simulink model "E3_1_Desequilibrio"  (R2018a)
settings: Solver=VariableStepAuto  StartTime=0.0  StopTime=0.5  RelTol=1e-3
libraries: powerlib x73, powerlib_meascontrol x36
settings Model: Creator=Rafael Pavan  LastModifiedBy=Rafael Pavan

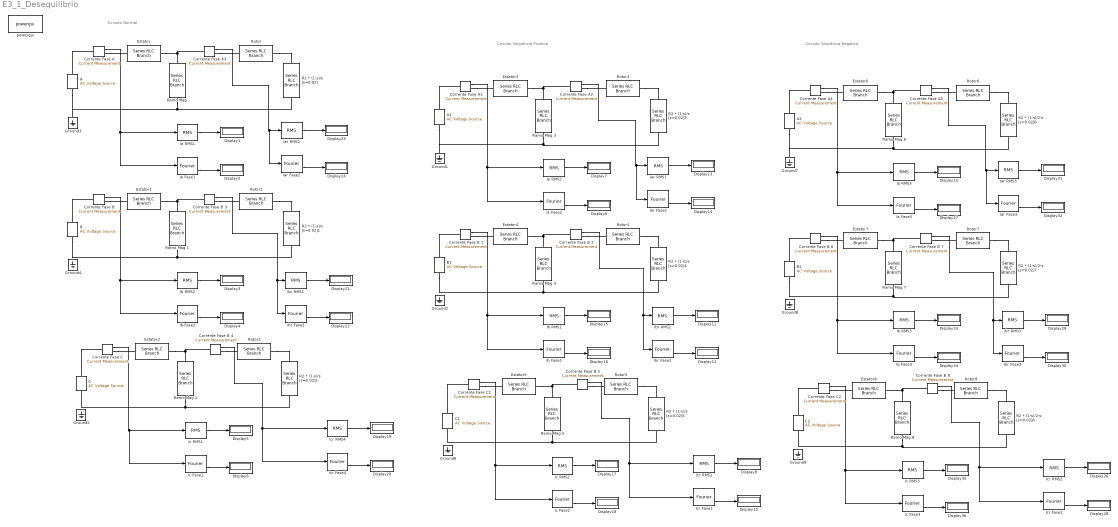
== system E3_1_Desequilibrio ==
  note: Circuito Normal
  note: Circuito Sequência Positiva
  note: Circuito Sequência Negativa
  A : powerlib/Electrical Sources/AC Voltage Source  Amplitude=171.26  Phase=0  Frequency=60  SampleTime=0  Measurements=None  BusType=PV  Pref=100e4  Qref=0  Qmin=-inf  Qmax=+inf
  A1 : powerlib/Electrical Sources/AC Voltage Source  Amplitude=179.5550  Phase=0  Frequency=60  SampleTime=0  Measurements=None  BusType=PV  Pref=100e4  Qref=0  Qmin=-inf  Qmax=+inf
  A2 : powerlib/Electrical Sources/AC Voltage Source  Amplitude=4.7693  Phase=-150.3406  Frequency=60  SampleTime=0  Measurements=None  BusType=PV  Pref=100e4  Qref=0  Qmin=-inf  Qmax=+inf
  B : powerlib/Electrical Sources/AC Voltage Source  Amplitude=179.605  Phase=-120  Frequency=60  SampleTime=0  Measurements=None  BusType=PV  Pref=100e4  Qref=0  Qmin=-inf  Qmax=+inf
  B1 : powerlib/Electrical Sources/AC Voltage Source  Amplitude=179.5550  Phase=-120  Frequency=60  SampleTime=0  Measurements=None  BusType=PV  Pref=100e4  Qref=0  Qmin=-inf  Qmax=+inf
  B2 : powerlib/Electrical Sources/AC Voltage Source  Amplitude=4.7693  Phase=-30.3441  Frequency=60  SampleTime=0  Measurements=None  BusType=PV  Pref=100e4  Qref=0  Qmin=-inf  Qmax=+inf
  C : powerlib/Electrical Sources/AC Voltage Source  Amplitude=187.80  Phase=120  Frequency=60  SampleTime=0  Measurements=None  BusType=PV  Pref=100e4  Qref=0  Qmin=-inf  Qmax=+inf
  C1 : powerlib/Electrical Sources/AC Voltage Source  Amplitude=179.5550  Phase=120  Frequency=60  SampleTime=0  Measurements=None  BusType=PV  Pref=100e4  Qref=0  Qmin=-inf  Qmax=+inf
  C2 : powerlib/Electrical Sources/AC Voltage Source  Amplitude=4.7693  Phase=89.6524  Frequency=60  SampleTime=0  Measurements=None  BusType=PV  Pref=100e4  Qref=0  Qmin=-inf  Qmax=+inf
  Corrente Fase A{,1..5} (6 alike) : powerlib/Measurements/Current Measurement  PhasorSimulation=off  OutputType=Complex  PSBequivalent=0
  Corrente Fase B {,1..8} (9 alike) : powerlib/Measurements/Current Measurement  PhasorSimulation=off  OutputType=Complex  PSBequivalent=0
  Corrente Fase C : powerlib/Measurements/Current Measurement  PhasorSimulation=off  OutputType=Complex  PSBequivalent=0
  Corrente Fase C1 : powerlib/Measurements/Current Measurement  PhasorSimulation=off  OutputType=Complex  PSBequivalent=0
  Corrente Fase C2 : powerlib/Measurements/Current Measurement  PhasorSimulation=off  OutputType=Complex  PSBequivalent=0
  Display{1..36} (36 alike) : Display
  Estator{,1..8} (9 alike) : powerlib/Elements/Series RLC Branch  LConnTagsString=__new0  RConnTagsString=__new0  BranchType=RL  Resistance=0.294  Inductance=1.33428e-3  SetiL0=off  InitialCurrent=0  Capacitance=1e-6  Setx0=off  InitialVoltage=0  Measurements=None
  Ground{1..9} (9 alike) : powerlib/Elements/Ground  LConnTagsString=a
  Ia Fase1 : powerlib_meascontrol/Measurements/Fourier  Freq=60  n=1  InInit=[0, 0]  Ts=0
      settings: SourceProductName=Simscape Power Systems
  Ia Fase2 : powerlib_meascontrol/Measurements/Fourier  Freq=60  n=1  InInit=[0, 0]  Ts=0
      settings: SourceProductName=Simscape Power Systems
  Ia Fase3 : powerlib_meascontrol/Measurements/Fourier  Freq=60  n=1  InInit=[0, 0]  Ts=0
      settings: SourceProductName=Simscape Power Systems
  Ia RMS1 : powerlib_meascontrol/Measurements/RMS  TrueRMS=on  Freq=60  RMSInit=120  Ts=0
  Ia RMS2 : powerlib_meascontrol/Measurements/RMS  TrueRMS=on  Freq=60  RMSInit=120  Ts=0
  Ia RMS3 : powerlib_meascontrol/Measurements/RMS  TrueRMS=on  Freq=60  RMSInit=120  Ts=0
  Iar Fase1 : powerlib_meascontrol/Measurements/Fourier  Freq=60  n=1  InInit=[0, 0]  Ts=0
      settings: SourceProductName=Simscape Power Systems
  Iar Fase2 : powerlib_meascontrol/Measurements/Fourier  Freq=60  n=1  InInit=[0, 0]  Ts=0
      settings: SourceProductName=Simscape Power Systems
  Iar Fase3 : powerlib_meascontrol/Measurements/Fourier  Freq=60  n=1  InInit=[0, 0]  Ts=0
      settings: SourceProductName=Simscape Power Systems
  Iar RMS1 : powerlib_meascontrol/Measurements/RMS  TrueRMS=on  Freq=60  RMSInit=120  Ts=0
  Iar RMS2 : powerlib_meascontrol/Measurements/RMS  TrueRMS=on  Freq=60  RMSInit=120  Ts=0
  Iar RMS3 : powerlib_meascontrol/Measurements/RMS  TrueRMS=on  Freq=60  RMSInit=120  Ts=0
  Ib Fase1 : powerlib_meascontrol/Measurements/Fourier  Freq=60  n=1  InInit=[0, 0]  Ts=0
      settings: SourceProductName=Simscape Power Systems
  Ib Fase2 : powerlib_meascontrol/Measurements/Fourier  Freq=60  n=1  InInit=[0, 0]  Ts=0
      settings: SourceProductName=Simscape Power Systems
  Ib Fase3 : powerlib_meascontrol/Measurements/Fourier  Freq=60  n=1  InInit=[0, 0]  Ts=0
      settings: SourceProductName=Simscape Power Systems
  Ib RMS1 : powerlib_meascontrol/Measurements/RMS  TrueRMS=on  Freq=60  RMSInit=120  Ts=0
  Ib RMS2 : powerlib_meascontrol/Measurements/RMS  TrueRMS=on  Freq=60  RMSInit=120  Ts=0
  Ib RMS3 : powerlib_meascontrol/Measurements/RMS  TrueRMS=on  Freq=60  RMSInit=120  Ts=0
  Ibr Fase1 : powerlib_meascontrol/Measurements/Fourier  Freq=60  n=1  InInit=[0, 0]  Ts=0
      settings: SourceProductName=Simscape Power Systems
  Ibr Fase2 : powerlib_meascontrol/Measurements/Fourier  Freq=60  n=1  InInit=[0, 0]  Ts=0
      settings: SourceProductName=Simscape Power Systems
  Ibr Fase3 : powerlib_meascontrol/Measurements/Fourier  Freq=60  n=1  InInit=[0, 0]  Ts=0
      settings: SourceProductName=Simscape Power Systems
  Ibr RMS1 : powerlib_meascontrol/Measurements/RMS  TrueRMS=on  Freq=60  RMSInit=120  Ts=0
  Ibr RMS2 : powerlib_meascontrol/Measurements/RMS  TrueRMS=on  Freq=60  RMSInit=120  Ts=0
  Ibr RMS3 : powerlib_meascontrol/Measurements/RMS  TrueRMS=on  Freq=60  RMSInit=120  Ts=0
  Ic Fase1 : powerlib_meascontrol/Measurements/Fourier  Freq=60  n=1  InInit=[0, 0]  Ts=0
      settings: SourceProductName=Simscape Power Systems
  Ic Fase2 : powerlib_meascontrol/Measurements/Fourier  Freq=60  n=1  InInit=[0, 0]  Ts=0
      settings: SourceProductName=Simscape Power Systems
  Ic Fase3 : powerlib_meascontrol/Measurements/Fourier  Freq=60  n=1  InInit=[0, 0]  Ts=0
      settings: SourceProductName=Simscape Power Systems
  Ic RMS1 : powerlib_meascontrol/Measurements/RMS  TrueRMS=on  Freq=60  RMSInit=120  Ts=0
  Ic RMS2 : powerlib_meascontrol/Measurements/RMS  TrueRMS=on  Freq=60  RMSInit=120  Ts=0
  Ic RMS3 : powerlib_meascontrol/Measurements/RMS  TrueRMS=on  Freq=60  RMSInit=120  Ts=0
  Icr Fase1 : powerlib_meascontrol/Measurements/Fourier  Freq=60  n=1  InInit=[0, 0]  Ts=0
      settings: SourceProductName=Simscape Power Systems
  Icr Fase2 : powerlib_meascontrol/Measurements/Fourier  Freq=60  n=1  InInit=[0, 0]  Ts=0
      settings: SourceProductName=Simscape Power Systems
  Icr Fase4 : powerlib_meascontrol/Measurements/Fourier  Freq=60  n=1  InInit=[0, 0]  Ts=0
      settings: SourceProductName=Simscape Power Systems
  Icr RMS1 : powerlib_meascontrol/Measurements/RMS  TrueRMS=on  Freq=60  RMSInit=120  Ts=0
  Icr RMS2 : powerlib_meascontrol/Measurements/RMS  TrueRMS=on  Freq=60  RMSInit=120  Ts=0
  Icr RMS4 : powerlib_meascontrol/Measurements/RMS  TrueRMS=on  Freq=60  RMSInit=120  Ts=0
  R2 * (1-s)/2-s [s=0.02]6 : powerlib/Elements/Series RLC Branch  LConnTagsString=__new0  RConnTagsString=__new0  BranchType=R  Resistance=0.2489  Inductance=1e-3  SetiL0=off  InitialCurrent=0  Capacitance=1e-6  Setx0=off  InitialVoltage=0  Measurements=None
  R2 * (1-s)/2-s [s=0.02]7 : powerlib/Elements/Series RLC Branch  LConnTagsString=__new0  RConnTagsString=__new0  BranchType=R  Resistance=0.2489  Inductance=1e-3  SetiL0=off  InitialCurrent=0  Capacitance=1e-6  Setx0=off  InitialVoltage=0  Measurements=None
  R2 * (1-s)/2-s [s=0.02]8 : powerlib/Elements/Series RLC Branch  LConnTagsString=__new0  RConnTagsString=__new0  BranchType=R  Resistance=0.2489  Inductance=1e-3  SetiL0=off  InitialCurrent=0  Capacitance=1e-6  Setx0=off  InitialVoltage=0  Measurements=None
  R2 * (1-s)/s [s=0.02]{,1..5} (6 alike) : powerlib/Elements/Series RLC Branch  LConnTagsString=__new0  RConnTagsString=__new0  BranchType=R  Resistance=24.647  Inductance=1e-3  SetiL0=off  InitialCurrent=0  Capacitance=1e-6  Setx0=off  InitialVoltage=0  Measurements=None
  Ramo Mag.{,1..8} (9 alike) : powerlib/Elements/Series RLC Branch  LConnTagsString=__new0  RConnTagsString=__new0  BranchType=L  Resistance=1  Inductance=0.0351477  SetiL0=off  InitialCurrent=0  Capacitance=1e-6  Setx0=off  InitialVoltage=0  Measurements=None
  Rotor{,1..8} (9 alike) : powerlib/Elements/Series RLC Branch  LConnTagsString=__new0  RConnTagsString=__new0  BranchType=RL  Resistance=0.503  Inductance=0.554406e-3  SetiL0=off  InitialCurrent=0  Capacitance=1e-6  Setx0=off  InitialVoltage=0  Measurements=None
  powergui : powerlib/powergui  Priority=1  SimulationMode=Continuous  SampleTime=50e-6  frequency=60  Iterations=50  frequencyindice=60  Pbase=100e6  ErrMax=1e-4  UnitsV=kV  UnitsW=MW  buscounter=0  FunctionMessages=on  echomessages=off  EnableUseOfTLC=off  CurrentSourceSwitches=off  DisableSnubberDevices=off  DisableRonSwitches=off  DisableVfSwitches=off  DisplayEquations=off  SolverType=Tustin/Backward Euler (TBE)  Interpol=off  ExternalGateDelay=off  methode=off  Ts=100  x0status=blocks  SPID=on  SwTol=0  HookPort=off  RestoreLinks=warning  ResistiveCurrentMeasurement=off  Frange=[0:2:500]  Ylog=off  Xlog=on  ShowGrid=off  save=off  variable=ZData  structure=0  ZoomFFT=off  StartTime=0.0  cycles=1  DisplayStyle=1  fundamental=60  FreqAxis=off  MaxFrequency=1000  frequencyindicesteady=1  RmsSteady=2  display=off
  wires:
  Ia RMS1/1 -> Display1/1
  Ia Fase1/2 -> Display2/1
  Corrente Fase A/1 -> Ia Fase1/1, Ia RMS1/1
  Ib RMS2/1 -> Display3/1
  Ib Fase2/2 -> Display4/1
  "Corrente Fase B "/1 -> Ib Fase2/1, Ib RMS2/1
  Corrente Fase C/1 -> Ic Fase1/1, Ic RMS1/1
  Ic Fase1/2 -> Display6/1
  Ic RMS1/1 -> Display5/1
  Corrente Fase B 4/1 -> Icr RMS4/1, Icr Fase4/1
  Icr Fase4/2 -> Display20/1
  Icr RMS4/1 -> Display19/1
  Ibr RMS1/1 -> Display21/1
  Ibr Fase1/2 -> Display22/1
  Corrente Fase B 3/1 -> Ibr RMS1/1, Ibr Fase1/1
  Iar Fase2/2 -> Display24/1
  Corrente Fase A3/1 -> Iar Fase2/1, Iar RMS2/1
  Iar RMS2/1 -> Display23/1
  Ib Fase1/2 -> Display16/1
  Ib RMS1/1 -> Display15/1
  Corrente Fase B 2/1 -> Ibr RMS2/1, Ibr Fase2/1
  Iar Fase1/2 -> Display14/1
  Ia Fase2/2 -> Display9/1
  Ic Fase2/2 -> Display18/1
  Corrente Fase C1/1 -> Ic Fase2/1, Ic RMS2/1
  Ibr RMS2/1 -> Display11/1
  Icr Fase1/2 -> Display10/1
  Iar RMS1/1 -> Display13/1
  Icr RMS1/1 -> Display8/1
  Corrente Fase B 1/1 -> Ib Fase1/1, Ib RMS1/1
  Ia RMS2/1 -> Display7/1
  Corrente Fase A2/1 -> Iar Fase1/1, Iar RMS1/1
  Ic RMS2/1 -> Display17/1
  Corrente Fase B 5/1 -> Icr RMS1/1, Icr Fase1/1
  Corrente Fase A1/1 -> Ia Fase2/1, Ia RMS2/1
  Ibr Fase2/2 -> Display12/1
  Ib Fase3/2 -> Display34/1
  Ib RMS3/1 -> Display33/1
  Corrente Fase B 7/1 -> Ibr RMS3/1, Ibr Fase3/1
  Iar Fase3/2 -> Display32/1
  Ia Fase3/2 -> Display27/1
  Ic Fase3/2 -> Display36/1
  Corrente Fase C2/1 -> Ic Fase3/1, Ic RMS3/1
  Ibr RMS3/1 -> Display29/1
  Icr Fase2/2 -> Display28/1
  Iar RMS3/1 -> Display31/1
  Icr RMS2/1 -> Display26/1
  Corrente Fase B 6/1 -> Ib Fase3/1, Ib RMS3/1
  Ia RMS3/1 -> Display25/1
  Corrente Fase A5/1 -> Iar Fase3/1, Iar RMS3/1
  Ic RMS3/1 -> Display35/1
  Corrente Fase B 8/1 -> Icr RMS2/1, Icr Fase2/1
  Corrente Fase A4/1 -> Ia Fase3/1, Ia RMS3/1
  Ibr Fase3/2 -> Display30/1
  connections:
  Estator/RConn1 -- Corrente Fase A3/LConn1 -- Ramo Mag./LConn1
  Rotor/RConn1 -- R2 * (1-s)/s [s=0.02]/LConn1
  Ramo Mag./RConn1 -- A/LConn1 -- Ground3/LConn1 -- R2 * (1-s)/s [s=0.02]/RConn1
  Corrente Fase A/RConn1 -- Estator/LConn1
  Corrente Fase A/LConn1 -- A/RConn1
  Estator1/RConn1 -- Corrente Fase B 3/LConn1 -- Ramo Mag.1/LConn1
  Ramo Mag.1/RConn1 -- B/LConn1 -- R2 * (1-s)/s [s=0.02]1/RConn1
  B/RConn1 -- "Corrente Fase B "/LConn1
  Rotor1/RConn1 -- R2 * (1-s)/s [s=0.02]1/LConn1
  "Corrente Fase B "/RConn1 -- Estator1/LConn1
  Estator2/RConn1 -- Corrente Fase B 4/LConn1 -- Ramo Mag.2/LConn1
  Ramo Mag.2/RConn1 -- C/LConn1 -- R2 * (1-s)/s [s=0.02]2/RConn1
  Corrente Fase C/RConn1 -- Estator2/LConn1
  Rotor2/RConn1 -- R2 * (1-s)/s [s=0.02]2/LConn1
  C/RConn1 -- Corrente Fase C/LConn1
  Corrente Fase A3/RConn1 -- Rotor/LConn1
  Corrente Fase B 3/RConn1 -- Rotor1/LConn1
  Corrente Fase B 4/RConn1 -- Rotor2/LConn1
  Ramo Mag.3/RConn1 -- R2 * (1-s)/s [s=0.02]3/RConn1 -- A1/LConn1 -- Ground1/LConn1
  Estator5/RConn1 -- Corrente Fase B 5/LConn1 -- Ramo Mag.5/LConn1
  Estator3/RConn1 -- Corrente Fase A2/LConn1 -- Ramo Mag.3/LConn1
  Ramo Mag.5/RConn1 -- C1/LConn1 -- R2 * (1-s)/s [s=0.02]5/RConn1
  Ramo Mag.4/RConn1 -- B1/LConn1 -- R2 * (1-s)/s [s=0.02]4/RConn1
  Estator4/RConn1 -- Corrente Fase B 2/LConn1 -- Ramo Mag.4/LConn1
  Rotor5/RConn1 -- R2 * (1-s)/s [s=0.02]5/LConn1
  Corrente Fase B 2/RConn1 -- Rotor4/LConn1
  C1/RConn1 -- Corrente Fase C1/LConn1
  B1/RConn1 -- Corrente Fase B 1/LConn1
  Corrente Fase B 5/RConn1 -- Rotor5/LConn1
  Corrente Fase B 1/RConn1 -- Estator4/LConn1
  Corrente Fase A2/RConn1 -- Rotor3/LConn1
  Corrente Fase C1/RConn1 -- Estator5/LConn1
  Corrente Fase A1/RConn1 -- Estator3/LConn1
  Rotor3/RConn1 -- R2 * (1-s)/s [s=0.02]3/LConn1
  Rotor4/RConn1 -- R2 * (1-s)/s [s=0.02]4/LConn1
  Corrente Fase A1/LConn1 -- A1/RConn1
  Ramo Mag.6/RConn1 -- R2 * (1-s)/2-s [s=0.02]6/RConn1 -- A2/LConn1 -- Ground7/LConn1
  Estator8/RConn1 -- Corrente Fase B 8/LConn1 -- Ramo Mag.8/LConn1
  Estator6/RConn1 -- Corrente Fase A5/LConn1 -- Ramo Mag.6/LConn1
  Ramo Mag.8/RConn1 -- C2/LConn1 -- R2 * (1-s)/2-s [s=0.02]8/RConn1
  Ramo Mag.7/RConn1 -- B2/LConn1 -- R2 * (1-s)/2-s [s=0.02]7/RConn1
  Estator7/RConn1 -- Corrente Fase B 7/LConn1 -- Ramo Mag.7/LConn1
  Rotor8/RConn1 -- R2 * (1-s)/2-s [s=0.02]8/LConn1
  Corrente Fase B 7/RConn1 -- Rotor7/LConn1
  C2/RConn1 -- Corrente Fase C2/LConn1
  B2/RConn1 -- Corrente Fase B 6/LConn1
  Corrente Fase B 8/RConn1 -- Rotor8/LConn1
  Corrente Fase B 6/RConn1 -- Estator7/LConn1
  Corrente Fase A5/RConn1 -- Rotor6/LConn1
  Corrente Fase C2/RConn1 -- Estator8/LConn1
  Corrente Fase A4/RConn1 -- Estator6/LConn1
  Rotor6/RConn1 -- R2 * (1-s)/2-s [s=0.02]6/LConn1
  Rotor7/RConn1 -- R2 * (1-s)/2-s [s=0.02]7/LConn1
  Corrente Fase A4/LConn1 -- A2/RConn1
